simulink model "wind_speed_test"  (R2014b)
settings: Solver=ode45  StartTime=0.0  StopTime=10  RelTol=1e-3
libraries: simulink x7
settings Model: Creator=daily_000  LastModifiedBy=daily_000

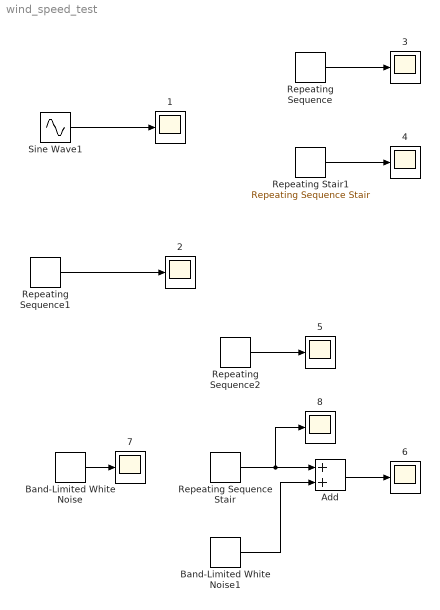
== system wind_speed_test ==
   {1..8} (8 alike) : Scope
      " 1" settings: YMin=2  YMax=4.5  SaveName=ScopeData12
      " 2" settings: YMin=2  YMax=4.5
      " 3" settings: YMin=2  YMax=4.5
      " 4" settings: YMin=2  YMax=4.5  SaveName=ScopeData2
      " 5" settings: YMin=2  YMax=4.5  SaveName=ScopeData3
      " 6" settings: YMin=2  YMax=4.5  SaveName=ScopeData4
      " 7" settings: YMin=2  YMax=4.5  SaveName=ScopeData5
      " 8" settings: YMin=2  YMax=4.5  SaveName=ScopeData6
  Add : Sum
  Band-Limited White Noise : simulink/Sources/Band-Limited White Noise  Cov=[0.001]  Ts=0.01  seed=[23341]
  Band-Limited White Noise1 : simulink/Sources/Band-Limited White Noise  Cov=[0.001]  Ts=0.01  seed=[23341]
  Repeating Sequence : simulink/Sources/Repeating Sequence  rep_seq_t=[0 2 3]  rep_seq_y=[0 5 1]
  Repeating Sequence Stair : simulink/Sources/Repeating Sequence Stair  OutValues=[0 2 3 2 1].'  tsamp=1  OutMin=[]  OutMax=[]  OutDataTypeStr=double  OutputDataTypeScalingMode=double  OutDataType=fixdt(0,8)  ConRadixGroup=Best Precision: Vector-wise  OutScaling=2^-12
  Repeating Sequence1 : simulink/Sources/Repeating Sequence  rep_seq_t=[0 5 7 10]  rep_seq_y=[4 9 6 4]
  Repeating Sequence2 : simulink/Sources/Repeating Sequence  rep_seq_t=[0 0.01 2 2.01 3]  rep_seq_y=[0 2 2 0 0]
  Repeating Stair1 : simulink/Sources/Repeating Sequence Stair  OutValues=[3 1 4 2 1].'  tsamp=-1  OutMin=[]  OutMax=[]  OutDataTypeStr=double  OutputDataTypeScalingMode=double  OutDataType=fixdt(0,8)  ConRadixGroup=Best Precision: Vector-wise  OutScaling=2^-12
  Sine Wave1 : Sin  Amplitude=5  Bias=4  Frequency=1/20*2*pi  SampleTime=0
  wires:
  Sine Wave1/1 -> " 1"/1
  Repeating Sequence1/1 -> " 2"/1
  Repeating Sequence/1 -> " 3"/1
  Repeating Stair1/1 -> " 4"/1
  Repeating Sequence2/1 -> " 5"/1
  Band-Limited White Noise/1 -> " 7"/1
  Repeating Sequence Stair/1 -> " 8"/1, Add/1
  Band-Limited White Noise1/1 -> Add/2
  Add/1 -> " 6"/1
